simulink model "ackerman_ROS_neural_controller_v2"  (R2023a)
settings: Solver=FixedStepDiscrete  StartTime=0.0  StopTime=200  FixedStep=0.1  RelTol=1e-3
undefined symbols (not defined in the file or in its folder): Angular, Linear
libraries: neural x413, robotlib x15, robotcorelib x1
(part 4 of 17)

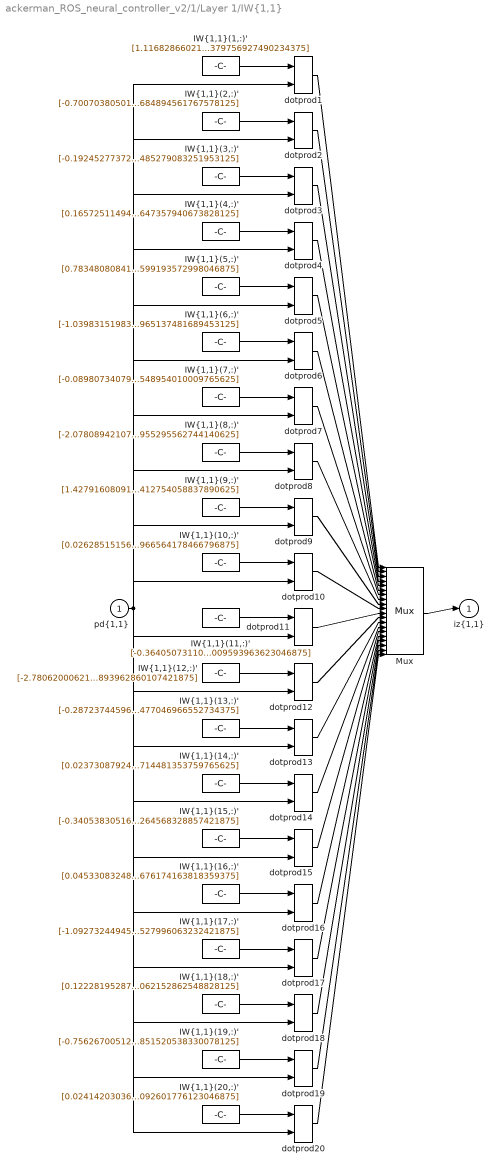
== system ackerman_ROS_neural_controller_v2/1/Layer 1/IW{1,1} ==
  "pd{1,1}" : Inport  PortDimensions=8  SampleTime=0.1
      mask Display: e = 0.06;c1 = [120 230 180]/255;c2 = ([120 230 180]+0)/(256+128);c3 = ([120 230 180]+128)/(256+128);patch([0 1 1 0],[0 0 1 1],c1);patch([0 1 1 1-e 1-e 0+e],[0 0 1 1-e 0+e 0+e],c2);patch([0 0 1 1-e 0+e 0+e],[0 1 1 1-e 1-e 0+e],c3);plot([0 1 1 0 0],[0 0 1 1 0]);
  "IW{1,1}(1,:)'" : Constant  Value=[1.116828660219907565220864853472448885440826416015625;-1.317372152173824861876028080587275326251983642578125;0.0888240780158889020601264974175137467682361602783203125;0.811843799445297609196359189809300005435943603515625;-0.0697394502326299237093820693189627490937709808349609375;-0.9124948278432263304438265549833886325359344482421875;0.48823599511569326647730804324964992702007293701171875;0.92312336239510184299206230207346379756927490234375]
      mask Display: e = 0.06;c1 = [120 150 230]/255;c2 = ([120 150 230]+0)/383;c3 = ([120 150 230]+128)/383;patch([0 1 1 0],[0 0 1 1],c1);patch([0 1 1 1-e 1-e 0+e],[0 0 1 1-e 0+e 0+e],c2);patch([0 0 1 1-e 0+e 0+e],[0 1 1 1-e 1-e 0+e],c3);plot([0 1 1 0 0],[0 0 1 1 0]);disp('Weights');
  "IW{1,1}(10,:)'" : Constant  Value=[0.0262851515602594322518203995286967256106436252593994140625;-2.5598472339347626558492265758104622364044189453125;-0.63500001320806076510194770889938808977603912353515625;0.08080628574030923605420184685499407351016998291015625;0.004282547131209214763547521442887955345213413238525390625;0.18751429268016039930699889737297780811786651611328125;0.50378156376655447434842471921001560986042022705078125;-0.52232179336882456066604163424926809966564178466796875]
      mask Display: e = 0.06;c1 = [120 150 230]/255;c2 = ([120 150 230]+0)/383;c3 = ([120 150 230]+128)/383;patch([0 1 1 0],[0 0 1 1],c1);patch([0 1 1 1-e 1-e 0+e],[0 0 1 1-e 0+e 0+e],c2);patch([0 0 1 1-e 0+e 0+e],[0 1 1 1-e 1-e 0+e],c3);plot([0 1 1 0 0],[0 0 1 1 0]);disp('Weights');
  "IW{1,1}(11,:)'" : Constant  Value=[-0.364050731103570779367828436079435050487518310546875;1.8340052162234459220968574300059117376804351806640625;0.0010169610273991704259277657484972223755903542041778564453125;0.58347480564712761452739187006955035030841827392578125;-0.9371891608231053272248800567467696964740753173828125;-0.721163434606463482623439631424844264984130859375;2.035079423445592450292451758286915719509124755859375;-0.34513579930387716654394125725957565009593963623046875]
      mask Display: e = 0.06;c1 = [120 150 230]/255;c2 = ([120 150 230]+0)/383;c3 = ([120 150 230]+128)/383;patch([0 1 1 0],[0 0 1 1],c1);patch([0 1 1 1-e 1-e 0+e],[0 0 1 1-e 0+e 0+e],c2);patch([0 0 1 1-e 0+e 0+e],[0 1 1 1-e 1-e 0+e],c3);plot([0 1 1 0 0],[0 0 1 1 0]);disp('Weights');
  "IW{1,1}(12,:)'" : Constant  Value=[-2.78062000621869831462618094519712030887603759765625;1.121862788646456277064089590567164123058319091796875;-1.8782585151834967351902605514624156057834625244140625;-1.8760642857863503163429186315624974668025970458984375;0.63081995495714615618254583750967867672443389892578125;1.7257064609143097921872822553268633782863616943359375;0.1502900196201445714994093805216834880411624908447265625;1.2290305602665305695353481496567837893962860107421875]
      mask Display: e = 0.06;c1 = [120 150 230]/255;c2 = ([120 150 230]+0)/383;c3 = ([120 150 230]+128)/383;patch([0 1 1 0],[0 0 1 1],c1);patch([0 1 1 1-e 1-e 0+e],[0 0 1 1-e 0+e 0+e],c2);patch([0 0 1 1-e 0+e 0+e],[0 1 1 1-e 1-e 0+e],c3);plot([0 1 1 0 0],[0 0 1 1 0]);disp('Weights');
  "IW{1,1}(13,:)'" : Constant  Value=[-0.2872374459617628161822722177021205425262451171875;-2.905786860043843233825100469402968883514404296875;-0.553996651955559027413755757152102887630462646484375;0.86810930276092801438636570310336537659168243408203125;-0.73141176276367680930690085006062872707843780517578125;0.687679406082589483872880009585060179233551025390625;0.1435056389676894472717805228967336006462574005126953125;-0.098326242430082311241079651153995655477046966552734375]
      mask Display: e = 0.06;c1 = [120 150 230]/255;c2 = ([120 150 230]+0)/383;c3 = ([120 150 230]+128)/383;patch([0 1 1 0],[0 0 1 1],c1);patch([0 1 1 1-e 1-e 0+e],[0 0 1 1-e 0+e 0+e],c2);patch([0 0 1 1-e 0+e 0+e],[0 1 1 1-e 1-e 0+e],c3);plot([0 1 1 0 0],[0 0 1 1 0]);disp('Weights');
  "IW{1,1}(14,:)'" : Constant  Value=[0.0237308792477848133628537397044055978767573833465576171875;-1.601784995976378578319554435438476502895355224609375;0.405350870218719183668554251198656857013702392578125;-0.007838045313262813340582368937248247675597667694091796875;0.32434432315157002424399479423300363123416900634765625;-1.0640785119557130133927103088353760540485382080078125;1.5009538196627640882496734775486402213573455810546875;-0.088510228652192657339270454031066037714481353759765625]
      mask Display: e = 0.06;c1 = [120 150 230]/255;c2 = ([120 150 230]+0)/383;c3 = ([120 150 230]+128)/383;patch([0 1 1 0],[0 0 1 1],c1);patch([0 1 1 1-e 1-e 0+e],[0 0 1 1-e 0+e 0+e],c2);patch([0 0 1 1-e 0+e 0+e],[0 1 1 1-e 1-e 0+e],c3);plot([0 1 1 0 0],[0 0 1 1 0]);disp('Weights');
  "IW{1,1}(15,:)'" : Constant  Value=[-0.3405383051671406757776594531605951488018035888671875;0.053295252358578293350177546017221175134181976318359375;1.035586391719500287678101813071407377719879150390625;1.923473416234176891492779759573750197887420654296875;-0.277425310964073024155851499017444439232349395751953125;-1.072290053858897973526609348482452332973480224609375;0.8387550177294522679716237689717672765254974365234375;-1.3760015689854945275527597914333455264568328857421875]
      mask Display: e = 0.06;c1 = [120 150 230]/255;c2 = ([120 150 230]+0)/383;c3 = ([120 150 230]+128)/383;patch([0 1 1 0],[0 0 1 1],c1);patch([0 1 1 1-e 1-e 0+e],[0 0 1 1-e 0+e 0+e],c2);patch([0 0 1 1-e 0+e 0+e],[0 1 1 1-e 1-e 0+e],c3);plot([0 1 1 0 0],[0 0 1 1 0]);disp('Weights');
  "IW{1,1}(16,:)'" : Constant  Value=[0.0453308324853925193043124863834236748516559600830078125;0.459559343539199749439916331539279781281948089599609375;-1.5227217158325867529811148415319621562957763671875;-0.6914425749720829461608673227601684629917144775390625;0.4436755063765982498580342507921159267425537109375;0.455038286792085522325379542962764389812946319580078125;0.9115280177617386403454702303861267864704132080078125;0.82498647477164011032613188945106230676174163818359375]
      mask Display: e = 0.06;c1 = [120 150 230]/255;c2 = ([120 150 230]+0)/383;c3 = ([120 150 230]+128)/383;patch([0 1 1 0],[0 0 1 1],c1);patch([0 1 1 1-e 1-e 0+e],[0 0 1 1-e 0+e 0+e],c2);patch([0 0 1 1-e 0+e 0+e],[0 1 1 1-e 1-e 0+e],c3);plot([0 1 1 0 0],[0 0 1 1 0]);disp('Weights');
  "IW{1,1}(17,:)'" : Constant  Value=[-1.0927324494595291870524533806019462645053863525390625;0.1538524822892356203052344199022627435624599456787109375;0.0671074562694427279030406907622818835079669952392578125;-0.57349675474466821345487232974846847355365753173828125;1.6003783061698844125686491679516620934009552001953125;1.60480486204609018585642843390814960002899169921875;-0.50380125898334504608300221661920659244060516357421875;0.59042401286813450678181425246293656527996063232421875]
      mask Display: e = 0.06;c1 = [120 150 230]/255;c2 = ([120 150 230]+0)/383;c3 = ([120 150 230]+128)/383;patch([0 1 1 0],[0 0 1 1],c1);patch([0 1 1 1-e 1-e 0+e],[0 0 1 1-e 0+e 0+e],c2);patch([0 0 1 1-e 0+e 0+e],[0 1 1 1-e 1-e 0+e],c3);plot([0 1 1 0 0],[0 0 1 1 0]);disp('Weights');
  "IW{1,1}(18,:)'" : Constant  Value=[0.12228195287823399872717544667466427199542522430419921875;-0.354406976130497763932680754805915057659149169921875;1.16787670361109707783953126636333763599395751953125;-0.171791758447963960332316446510958485305309295654296875;-0.7120100985359341105862540644011460244655609130859375;-1.0292471435836361148830064848880283534526824951171875;-1.6915065806122473457406840680050663650035858154296875;0.2143675751442244703515171977414865978062152862548828125]
      mask Display: e = 0.06;c1 = [120 150 230]/255;c2 = ([120 150 230]+0)/383;c3 = ([120 150 230]+128)/383;patch([0 1 1 0],[0 0 1 1],c1);patch([0 1 1 1-e 1-e 0+e],[0 0 1 1-e 0+e 0+e],c2);patch([0 0 1 1-e 0+e 0+e],[0 1 1 1-e 1-e 0+e],c3);plot([0 1 1 0 0],[0 0 1 1 0]);disp('Weights');
  "IW{1,1}(19,:)'" : Constant  Value=[-0.7562670051233231216514241168624721467494964599609375;-0.85460135528397873638795090300845913589000701904296875;0.85019606027952299154293314131791703402996063232421875;0.1161628518467531512303736462854431010782718658447265625;-1.0109441109467194319648797318222932517528533935546875;-0.94125834497824223401352128348662517964839935302734375;-0.794270812434147988057020484120585024356842041015625;-0.3913546009844559581125622571562416851520538330078125]
      mask Display: e = 0.06;c1 = [120 150 230]/255;c2 = ([120 150 230]+0)/383;c3 = ([120 150 230]+128)/383;patch([0 1 1 0],[0 0 1 1],c1);patch([0 1 1 1-e 1-e 0+e],[0 0 1 1-e 0+e 0+e],c2);patch([0 0 1 1-e 0+e 0+e],[0 1 1 1-e 1-e 0+e],c3);plot([0 1 1 0 0],[0 0 1 1 0]);disp('Weights');
  "IW{1,1}(2,:)'" : Constant  Value=[-0.70070380501134021944409369098138995468616485595703125;0.4463782749714180209110736541333608329296112060546875;0.67982390187422991889576451285392977297306060791015625;-0.66805266049382705517700742348097264766693115234375;0.65873385787125737778069378691725432872772216796875;0.80873570737898192728465573964058421552181243896484375;1.607933726033231369711984370951540768146514892578125;0.0282312561074684886808228156951372511684894561767578125]
      mask Display: e = 0.06;c1 = [120 150 230]/255;c2 = ([120 150 230]+0)/383;c3 = ([120 150 230]+128)/383;patch([0 1 1 0],[0 0 1 1],c1);patch([0 1 1 1-e 1-e 0+e],[0 0 1 1-e 0+e 0+e],c2);patch([0 0 1 1-e 0+e 0+e],[0 1 1 1-e 1-e 0+e],c3);plot([0 1 1 0 0],[0 0 1 1 0]);disp('Weights');
  "IW{1,1}(20,:)'" : Constant  Value=[0.0241420303636170376082592525790460058487951755523681640625;-0.222720935580721646207535968642332591116428375244140625;0.323902677318082365953699763849726878106594085693359375;-0.6235037611809357560588296109926886856555938720703125;-0.69145330685383232793839169971761293709278106689453125;-1.0351207523282039968393064555129967629909515380859375;0.365678623892759235847194076995947398245334625244140625;-2.616536737179383731444204386207275092601776123046875]
      mask Display: e = 0.06;c1 = [120 150 230]/255;c2 = ([120 150 230]+0)/383;c3 = ([120 150 230]+128)/383;patch([0 1 1 0],[0 0 1 1],c1);patch([0 1 1 1-e 1-e 0+e],[0 0 1 1-e 0+e 0+e],c2);patch([0 0 1 1-e 0+e 0+e],[0 1 1 1-e 1-e 0+e],c3);plot([0 1 1 0 0],[0 0 1 1 0]);disp('Weights');
  "IW{1,1}(3,:)'" : Constant  Value=[-0.1924527737266698290685695837964885868132114410400390625;-0.98526738913007749776085120174684561789035797119140625;1.182387309836708144672456910484470427036285400390625;0.140201368902994116805160729199997149407863616943359375;-1.784628432745574588835779650253243744373321533203125;0.8833279993245153338676800558459945023059844970703125;0.8505388438650627325188224858720786869525909423828125;-0.331496701624171496991522190000978298485279083251953125]
      mask Display: e = 0.06;c1 = [120 150 230]/255;c2 = ([120 150 230]+0)/383;c3 = ([120 150 230]+128)/383;patch([0 1 1 0],[0 0 1 1],c1);patch([0 1 1 1-e 1-e 0+e],[0 0 1 1-e 0+e 0+e],c2);patch([0 0 1 1-e 0+e 0+e],[0 1 1 1-e 1-e 0+e],c3);plot([0 1 1 0 0],[0 0 1 1 0]);disp('Weights');
  "IW{1,1}(4,:)'" : Constant  Value=[0.1657251149471581086469740284883300773799419403076171875;0.11079163994764328060593783220610930584371089935302734375;1.1628412946805528616067704206216149032115936279296875;1.3120470595789817114251718521700240671634674072265625;0.5705449810256768561345097623416222631931304931640625;0.2195264626413448161290631333031342364847660064697265625;-2.660419563695247457957293590879999101161956787109375;-0.7954052280397139185197374899871647357940673828125]
      mask Display: e = 0.06;c1 = [120 150 230]/255;c2 = ([120 150 230]+0)/383;c3 = ([120 150 230]+128)/383;patch([0 1 1 0],[0 0 1 1],c1);patch([0 1 1 1-e 1-e 0+e],[0 0 1 1-e 0+e 0+e],c2);patch([0 0 1 1-e 0+e 0+e],[0 1 1 1-e 1-e 0+e],c3);plot([0 1 1 0 0],[0 0 1 1 0]);disp('Weights');
  "IW{1,1}(5,:)'" : Constant  Value=[0.7834808084145892248528753043501637876033782958984375;-1.42447445469726829969658865593373775482177734375;1.1975312359302596743049207361764274537563323974609375;0.1635490607498303050615362508324324153363704681396484375;-0.6718969042920146517161583687993697822093963623046875;-0.1372657172031984396110004809088422916829586029052734375;0.38125925588003173327678041459876112639904022216796875;-1.4402596893604620031936747182044200599193572998046875]
      mask Display: e = 0.06;c1 = [120 150 230]/255;c2 = ([120 150 230]+0)/383;c3 = ([120 150 230]+128)/383;patch([0 1 1 0],[0 0 1 1],c1);patch([0 1 1 1-e 1-e 0+e],[0 0 1 1-e 0+e 0+e],c2);patch([0 0 1 1-e 0+e 0+e],[0 1 1 1-e 1-e 0+e],c3);plot([0 1 1 0 0],[0 0 1 1 0]);disp('Weights');
  "IW{1,1}(6,:)'" : Constant  Value=[-1.0398315198302390260920446962700225412845611572265625;1.0759366572930788574780081034987233579158782958984375;-0.180033990146306888124883016644162125885486602783203125;-1.348012567824036889163608066155575215816497802734375;-2.885573301576848326277513478999026119709014892578125;-0.2948558223190076432729256339371204376220703125;1.2807460752471115927875189299811609089374542236328125;0.08268843179290515099655323183469590730965137481689453125]
      mask Display: e = 0.06;c1 = [120 150 230]/255;c2 = ([120 150 230]+0)/383;c3 = ([120 150 230]+128)/383;patch([0 1 1 0],[0 0 1 1],c1);patch([0 1 1 1-e 1-e 0+e],[0 0 1 1-e 0+e 0+e],c2);patch([0 0 1 1-e 0+e 0+e],[0 1 1 1-e 1-e 0+e],c3);plot([0 1 1 0 0],[0 0 1 1 0]);disp('Weights');
  "IW{1,1}(7,:)'" : Constant  Value=[-0.08980734079662848479141956659077550284564495086669921875;-0.1641338178963755167760751874084235168993473052978515625;0.405589455292452161216942840837873518466949462890625;1.076734142043771047525524409138597548007965087890625;0.54123529493598188100378365561482496559619903564453125;1.1029221929994712514400134750758297741413116455078125;1.648597514590885548813048444571904838085174560546875;-1.5057803317372295826004346963600255548954010009765625]
      mask Display: e = 0.06;c1 = [120 150 230]/255;c2 = ([120 150 230]+0)/383;c3 = ([120 150 230]+128)/383;patch([0 1 1 0],[0 0 1 1],c1);patch([0 1 1 1-e 1-e 0+e],[0 0 1 1-e 0+e 0+e],c2);patch([0 0 1 1-e 0+e 0+e],[0 1 1 1-e 1-e 0+e],c3);plot([0 1 1 0 0],[0 0 1 1 0]);disp('Weights');
  "IW{1,1}(8,:)'" : Constant  Value=[-2.07808942107180172342850710265338420867919921875;-1.0129688078326017919295054525719024240970611572265625;0.275033497576107344162466006309841759502887725830078125;0.48072637579094390503087197430431842803955078125;-0.023912142949013927284429570363499806262552738189697265625;0.5059355504927471880449729724205099046230316162109375;-0.46415439958115023433293799826060421764850616455078125;2.02330328464420805545387338497675955295562744140625]
      mask Display: e = 0.06;c1 = [120 150 230]/255;c2 = ([120 150 230]+0)/383;c3 = ([120 150 230]+128)/383;patch([0 1 1 0],[0 0 1 1],c1);patch([0 1 1 1-e 1-e 0+e],[0 0 1 1-e 0+e 0+e],c2);patch([0 0 1 1-e 0+e 0+e],[0 1 1 1-e 1-e 0+e],c3);plot([0 1 1 0 0],[0 0 1 1 0]);disp('Weights');
  "IW{1,1}(9,:)'" : Constant  Value=[1.4279160809158355505132931284606456756591796875;-1.035532835891061598232454343815334141254425048828125;-0.5968860108683367027282429262413643300533294677734375;-1.2494838793611282579121279923128895461559295654296875;3.934956615032649818175514155882410705089569091796875;0.1307241221935328268077824986903578974306583404541015625;-2.457926598366699355580067276605404913425445556640625;-1.627164141237702921216623508371412754058837890625]
      mask Display: e = 0.06;c1 = [120 150 230]/255;c2 = ([120 150 230]+0)/383;c3 = ([120 150 230]+128)/383;patch([0 1 1 0],[0 0 1 1],c1);patch([0 1 1 1-e 1-e 0+e],[0 0 1 1-e 0+e 0+e],c2);patch([0 0 1 1-e 0+e 0+e],[0 1 1 1-e 1-e 0+e],c3);plot([0 1 1 0 0],[0 0 1 1 0]);disp('Weights');
  Mux : Mux  Inputs=20
      mask Display: e = 0.06;c1 = [120 150 230]/255;c2 = ([120 150 230]+0)/383;c3 = ([120 150 230]+128)/383;patch([0 1 1 0],[0 0 1 1],c1);patch([0 1 1 1-e 1-e 0+e],[0 0 1 1-e 0+e 0+e],c2);patch([0 0 1 1-e 0+e 0+e],[0 1 1 1-e 1-e 0+e],c3);plot([0 1 1 0 0],[0 0 1 1 0]);disp('Mux');
  dotprod{1..20} (20 alike) : neural/Weight Functions/dotprod
  "iz{1,1}" : Outport
      mask Display: e = 0.06;c1 = [120 230 180]/255;c2 = ([120 230 180]+0)/(256+128);c3 = ([120 230 180]+128)/(256+128);patch([0 1 1 0],[0 0 1 1],c1);patch([0 1 1 1-e 1-e 0+e],[0 0 1 1-e 0+e 0+e],c2);patch([0 0 1 1-e 0+e 0+e],[0 1 1 1-e 1-e 0+e],c3);plot([0 1 1 0 0],[0 0 1 1 0]);
  wires:
  "IW{1,1}(1,:)'"/1 -> dotprod1/1
  "pd{1,1}"/1 -> dotprod1/2, dotprod2/2, dotprod3/2, dotprod4/2, dotprod5/2, dotprod6/2, dotprod7/2, dotprod8/2, dotprod9/2, dotprod10/2, dotprod11/2, dotprod12/2, dotprod13/2, dotprod14/2, dotprod15/2, dotprod16/2, dotprod17/2, dotprod18/2, dotprod19/2, dotprod20/2
  dotprod1/1 -> Mux/1
  "IW{1,1}(2,:)'"/1 -> dotprod2/1
  dotprod2/1 -> Mux/2
  "IW{1,1}(3,:)'"/1 -> dotprod3/1
  dotprod3/1 -> Mux/3
  "IW{1,1}(4,:)'"/1 -> dotprod4/1
  dotprod4/1 -> Mux/4
  "IW{1,1}(5,:)'"/1 -> dotprod5/1
  dotprod5/1 -> Mux/5
  "IW{1,1}(6,:)'"/1 -> dotprod6/1
  dotprod6/1 -> Mux/6
  "IW{1,1}(7,:)'"/1 -> dotprod7/1
  dotprod7/1 -> Mux/7
  "IW{1,1}(8,:)'"/1 -> dotprod8/1
  dotprod8/1 -> Mux/8
  "IW{1,1}(9,:)'"/1 -> dotprod9/1
  dotprod9/1 -> Mux/9
  "IW{1,1}(10,:)'"/1 -> dotprod10/1
  dotprod10/1 -> Mux/10
  "IW{1,1}(11,:)'"/1 -> dotprod11/1
  dotprod11/1 -> Mux/11
  "IW{1,1}(12,:)'"/1 -> dotprod12/1
  dotprod12/1 -> Mux/12
  "IW{1,1}(13,:)'"/1 -> dotprod13/1
  dotprod13/1 -> Mux/13
  "IW{1,1}(14,:)'"/1 -> dotprod14/1
  dotprod14/1 -> Mux/14
  "IW{1,1}(15,:)'"/1 -> dotprod15/1
  dotprod15/1 -> Mux/15
  "IW{1,1}(16,:)'"/1 -> dotprod16/1
  dotprod16/1 -> Mux/16
  "IW{1,1}(17,:)'"/1 -> dotprod17/1
  dotprod17/1 -> Mux/17
  "IW{1,1}(18,:)'"/1 -> dotprod18/1
  dotprod18/1 -> Mux/18
  "IW{1,1}(19,:)'"/1 -> dotprod19/1
  dotprod19/1 -> Mux/19
  "IW{1,1}(20,:)'"/1 -> dotprod20/1
  dotprod20/1 -> Mux/20
  Mux/1 -> "iz{1,1}"/1

== system ackerman_ROS_neural_controller_v2/1/Layer 2/Delays 1 ==
  "p{2}" : Inport  PortDimensions=20  SampleTime=0.1
      mask Display: e = 0.06;c1 = [120 230 180]/255;c2 = ([120 230 180]+0)/(256+128);c3 = ([120 230 180]+128)/(256+128);patch([0 1 1 0],[0 0 1 1],c1);patch([0 1 1 1-e 1-e 0+e],[0 0 1 1-e 0+e 0+e],c2);patch([0 0 1 1-e 0+e 0+e],[0 1 1 1-e 1-e 0+e],c3);plot([0 1 1 0 0],[0 0 1 1 0]);
  mux : Mux  Inputs=1
      mask Display: e = 0.06;c1 = [120 150 230]/255;c2 = ([120 150 230]+0)/383;c3 = ([120 150 230]+128)/383;patch([0 1 1 0],[0 0 1 1],c1);patch([0 1 1 1-e 1-e 0+e],[0 0 1 1-e 0+e 0+e],c2);patch([0 0 1 1-e 0+e 0+e],[0 1 1 1-e 1-e 0+e],c3);plot([0 1 1 0 0],[0 0 1 1 0]);disp('Mux')
  "pd{2,1}" : Outport
      mask Display: e = 0.06;c1 = [120 230 180]/255;c2 = ([120 230 180]+0)/(256+128);c3 = ([120 230 180]+128)/(256+128);patch([0 1 1 0],[0 0 1 1],c1);patch([0 1 1 1-e 1-e 0+e],[0 0 1 1-e 0+e 0+e],c2);patch([0 0 1 1-e 0+e 0+e],[0 1 1 1-e 1-e 0+e],c3);plot([0 1 1 0 0],[0 0 1 1 0]);
  wires:
  "p{2}"/1 -> mux/1
  mux/1 -> "pd{2,1}"/1

== system ackerman_ROS_neural_controller_v2/1/Layer 2/LW{2,1} ==
  "ad{2,1}" : Inport  PortDimensions=20  SampleTime=0.1
      mask Display: e = 0.06;c1 = [120 230 180]/255;c2 = ([120 230 180]+0)/(256+128);c3 = ([120 230 180]+128)/(256+128);patch([0 1 1 0],[0 0 1 1],c1);patch([0 1 1 1-e 1-e 0+e],[0 0 1 1-e 0+e 0+e],c2);patch([0 0 1 1-e 0+e 0+e],[0 1 1 1-e 1-e 0+e],c3);plot([0 1 1 0 0],[0 0 1 1 0]);
  "IW{2,1}(1,:)'" : Constant  Value=[0.110281640354253307467757849735789932310581207275390625;-0.4075499594610167974906289600767195224761962890625;-0.211945196756619658184916943355347029864788055419921875;-1.0447559407086106642026379631715826690196990966796875;0.99973827271722426335287536858231760561466217041015625;1.1187491991695612814083915509399957954883575439453125;-0.8574904128367728528559155165567062795162200927734375;-1.9045319663374866703264842726639471948146820068359375;2.507081512845534376765499473549425601959228515625;0.0009773874370581879522656976178041077218949794769287109375;0.1290398987580549661213780154866981320083141326904296875;-0.884324725107169751225910658831708133220672607421875;-0.448646363139221182603222359830397181212902069091796875;-0.5078166421618230952361727759125642478466033935546875;-1.0801208830190149878802685634582303464412689208984375;-0.220075278352753922472828662648680619895458221435546875;0.1932052062463338604203499926370568573474884033203125;-0.268976457076010866398263488008524291217327117919921875;0.8706129490286713679125796261359937489032745361328125;-0.12354111103369637414406412290190928615629673004150390625]
      mask Display: e = 0.06;c1 = [120 150 230]/255;c2 = ([120 150 230]+0)/383;c3 = ([120 150 230]+128)/383;patch([0 1 1 0],[0 0 1 1],c1);patch([0 1 1 1-e 1-e 0+e],[0 0 1 1-e 0+e 0+e],c2);patch([0 0 1 1-e 0+e 0+e],[0 1 1 1-e 1-e 0+e],c3);plot([0 1 1 0 0],[0 0 1 1 0]);disp('weights');
  "IW{2,1}(10,:)'" : Constant  Value=[0.346280781819803429311122044964577071368694305419921875;0.064764388127894034763443187330267392098903656005859375;-0.198841117778091935885953489560051821172237396240234375;-0.1526219736868450194133828290432575158774852752685546875;-0.315671952489745388792385938359075225889682769775390625;0.41149032816694230962895062475581653416156768798828125;0.179963111618439197680885399677208624780178070068359375;-0.6692435375154885957016404063324443995952606201171875;-0.69612096619450680723417690387577749788761138916015625;-0.42825439692942079972226565587334334850311279296875;0.041563970098095683047834114631768898107111454010009765625;-0.1601867703146730714802714601319166831672191619873046875;0.6738085909001958473396598492399789392948150634765625;0.1940185562231697968815780086515587754547595977783203125;-0.342702712650292451446176755780470557510852813720703125;0.74770586496094837425374635131447575986385345458984375;-0.25702064669828994514233500012778677046298980712890625;0.31617480897826855112953126081265509128570556640625;-0.24096465028794700202752210316248238086700439453125;-0.7483797507369989165937340658274479210376739501953125]
      mask Display: e = 0.06;c1 = [120 150 230]/255;c2 = ([120 150 230]+0)/383;c3 = ([120 150 230]+128)/383;patch([0 1 1 0],[0 0 1 1],c1);patch([0 1 1 1-e 1-e 0+e],[0 0 1 1-e 0+e 0+e],c2);patch([0 0 1 1-e 0+e 0+e],[0 1 1 1-e 1-e 0+e],c3);plot([0 1 1 0 0],[0 0 1 1 0]);disp('weights');
  "IW{2,1}(2,:)'" : Constant  Value=[-0.3144161658093695965732194963493384420871734619140625;-0.260802005499317868242314943927340209484100341796875;-0.09118866387487238600595418347438680939376354217529296875;-0.1779746583379019087001182697349577210843563079833984375;0.273944070348914270329743203546968288719654083251953125;0.1429879515740476170204686923170811496675014495849609375;-0.353011636830328157099501140692154876887798309326171875;-0.48203732900629636670686295474297367036342620849609375;-0.5762308390680572767195144479046575725078582763671875;-0.147680072840977005821372358695953153073787689208984375;-0.351694320118391690055403842052328400313854217529296875;-0.12110239440517685249876222997045260854065418243408203125;-0.1729993563477275342332717400495312176644802093505859375;-0.2449324314496446886035840861950418911874294281005859375;0.290852554535415308567536385453422553837299346923828125;0.48214156352169867947310422096052207052707672119140625;-0.1768665440642207264954066658901865594089031219482421875;-0.6433962295717943202788546841475181281566619873046875;-0.61118602203887972823537211297661997377872467041015625;-0.64264309517045792308209684051689691841602325439453125]
      mask Display: e = 0.06;c1 = [120 150 230]/255;c2 = ([120 150 230]+0)/383;c3 = ([120 150 230]+128)/383;patch([0 1 1 0],[0 0 1 1],c1);patch([0 1 1 1-e 1-e 0+e],[0 0 1 1-e 0+e 0+e],c2);patch([0 0 1 1-e 0+e 0+e],[0 1 1 1-e 1-e 0+e],c3);plot([0 1 1 0 0],[0 0 1 1 0]);disp('weights');
  "IW{2,1}(3,:)'" : Constant  Value=[-1.0531416570213278927070632562390528619289398193359375;0.021168604966173142079011171290403581224381923675537109375;-0.497619065788888426116187702064053155481815338134765625;-0.70600061911108136225578846278949640691280364990234375;-0.799145216720182904879266061470843851566314697265625;0.656441274846339073434364763670600950717926025390625;-1.0986685679554508698885229023289866745471954345703125;0.5647820076666738575710269287810660898685455322265625;1.2692212929800776866073874771245755255222320556640625;0.400332946434238723387721847757347859442234039306640625;-0.1089433289215561428964207379976869560778141021728515625;-1.818493460995366017840524364146403968334197998046875;-0.66180348114890608091087642605998553335666656494140625;-1.2170049059022656212647461870801635086536407470703125;0.8486535437562900963115453123464249074459075927734375;0.37739936148836650264826175771304406225681304931640625;1.2761023790039784930883115521282888948917388916015625;-1.396101663000505421763364211074076592922210693359375;0.05986777040123077153754849177857977338135242462158203125;-0.1085682225433008130099921118016936816275119781494140625]
      mask Display: e = 0.06;c1 = [120 150 230]/255;c2 = ([120 150 230]+0)/383;c3 = ([120 150 230]+128)/383;patch([0 1 1 0],[0 0 1 1],c1);patch([0 1 1 1-e 1-e 0+e],[0 0 1 1-e 0+e 0+e],c2);patch([0 0 1 1-e 0+e 0+e],[0 1 1 1-e 1-e 0+e],c3);plot([0 1 1 0 0],[0 0 1 1 0]);disp('weights');
  "IW{2,1}(4,:)'" : Constant  Value=[0.7802649519735174177270664586103521287441253662109375;-0.2171648780590997585004942038722219876945018768310546875;-0.2644108571941050644937831748393364250659942626953125;-0.2326443889087644045776670509440009482204914093017578125;-1.443034579947640505537265198654495179653167724609375;-1.650885089865213206650196298141963779926300048828125;0.5932390807268961285814157236018218100070953369140625;-0.423310015863895883203582570786238647997379302978515625;-0.7824745148668592609197958154254592955112457275390625;-1.0564054180223629852974909226759336888790130615234375;-0.48060704625918904131509634680696763098239898681640625;0.394917352231212548385741456513642333447933197021484375;-1.6965769318066958870616645072004757821559906005859375;-0.82689983880989059716881683925748802721500396728515625;-0.66916391659144658365931945809279568493366241455078125;-0.334444529874724338913694055008818395435810089111328125;-1.65208126900715246421214033034630119800567626953125;1.364022987750377335913753995555453002452850341796875;-0.0093443227721153702958201137107607792131602764129638671875;-0.56926038307607884636496464736410416662693023681640625]
      mask Display: e = 0.06;c1 = [120 150 230]/255;c2 = ([120 150 230]+0)/383;c3 = ([120 150 230]+128)/383;patch([0 1 1 0],[0 0 1 1],c1);patch([0 1 1 1-e 1-e 0+e],[0 0 1 1-e 0+e 0+e],c2);patch([0 0 1 1-e 0+e 0+e],[0 1 1 1-e 1-e 0+e],c3);plot([0 1 1 0 0],[0 0 1 1 0]);disp('weights');
  "IW{2,1}(5,:)'" : Constant  Value=[-1.69558095268002251287953185965307056903839111328125;-0.036402227108619421291901829818016267381608486175537109375;0.79510630105207347195772626946563832461833953857421875;1.288678002327857452513626412837766110897064208984375;0.50338188136540684691766500691301189363002777099609375;0.0718388753007755120894017863975022919476032257080078125;0.89626959568035380332418071702704764902591705322265625;-1.545785879539742335708751852507703006267547607421875;-0.94793395213213982319899741924018599092960357666015625;1.225767400049665223349393272656016051769256591796875;-0.1410385296484627792867883044891641475260257720947265625;-2.26987855069070310065626472351141273975372314453125;0.82063433795832640971212867952999658882617950439453125;0.5657515729250663927274445086368359625339508056640625;1.474012242783430348680440147290937602519989013671875;0.638039091111959777435913565568625926971435546875;-0.6381713375893458550791592642781324684619903564453125;-1.1708364908966777395704639275209046900272369384765625;-0.19528457479245509009757597596035338938236236572265625;-0.6839118851799159681803530475008301436901092529296875]
      mask Display: e = 0.06;c1 = [120 150 230]/255;c2 = ([120 150 230]+0)/383;c3 = ([120 150 230]+128)/383;patch([0 1 1 0],[0 0 1 1],c1);patch([0 1 1 1-e 1-e 0+e],[0 0 1 1-e 0+e 0+e],c2);patch([0 0 1 1-e 0+e 0+e],[0 1 1 1-e 1-e 0+e],c3);plot([0 1 1 0 0],[0 0 1 1 0]);disp('weights');
  "IW{2,1}(6,:)'" : Constant  Value=[0.323379113562345665844333097993512637913227081298828125;0.63603235307997330050255868627573363482952117919921875;0.9136038407711459807813980660284869372844696044921875;-0.56666095330895605020060656897840090095996856689453125;0.159876383499391316878046609417651779949665069580078125;0.62063551392938454132064407531288452446460723876953125;0.2516353424530215487919804218108765780925750732421875;-0.104656037316503469636330692082992754876613616943359375;2.097313473759132573803753984975628554821014404296875;0.07834531276352570128285179862359655089676380157470703125;2.195634643091262550029796329909004271030426025390625;-1.3286965266555343934129496119567193090915679931640625;1.46608549856063330452116133528761565685272216796875;-0.88004902451046318478944385788054205477237701416015625;0.7740781740302422608834831407875753939151763916015625;-0.37138408893100860463931667254655621945858001708984375;1.604442288304878783122831009677611291408538818359375;-0.449110542112181210239185702448594383895397186279296875;0.06659377782630350461889889857047819532454013824462890625;-0.6823935781906842468202967211254872381687164306640625]
      mask Display: e = 0.06;c1 = [120 150 230]/255;c2 = ([120 150 230]+0)/383;c3 = ([120 150 230]+128)/383;patch([0 1 1 0],[0 0 1 1],c1);patch([0 1 1 1-e 1-e 0+e],[0 0 1 1-e 0+e 0+e],c2);patch([0 0 1 1-e 0+e 0+e],[0 1 1 1-e 1-e 0+e],c3);plot([0 1 1 0 0],[0 0 1 1 0]);disp('weights');
  "IW{2,1}(7,:)'" : Constant  Value=[0.32539695260053724812365771867916919291019439697265625;1.0963993598379910832107952955993823707103729248046875;-1.330554666607169256309362026513554155826568603515625;0.442056302963367897529423089508782140910625457763671875;0.82216341442806761818928862339816987514495849609375;-0.30352716797758072519997085692011751234531402587890625;0.2136723848484809451520050060935318470001220703125;-0.84521000613493135755760476968134753406047821044921875;-0.474420040044124025069294248169171623885631561279296875;-0.65302179764648382587211017380468547344207763671875;-0.106792482967198620880111548103741370141506195068359375;-0.004261715654998519953178259811465977691113948822021484375;-0.45342284495086493389948145704693160951137542724609375;-0.44167171573887176183603742174454964697360992431640625;0.054384844545579659469414224304273375310003757476806640625;-0.2631948573202540497817381037748418748378753662109375;-0.91589517807826392736814113959553651511669158935546875;-0.298081126093376891361685920855961740016937255859375;-0.00160608898792290850053576800604560048668645322322845458984375;-0.7363276965989420386193842205102555453777313232421875]
      mask Display: e = 0.06;c1 = [120 150 230]/255;c2 = ([120 150 230]+0)/383;c3 = ([120 150 230]+128)/383;patch([0 1 1 0],[0 0 1 1],c1);patch([0 1 1 1-e 1-e 0+e],[0 0 1 1-e 0+e 0+e],c2);patch([0 0 1 1-e 0+e 0+e],[0 1 1 1-e 1-e 0+e],c3);plot([0 1 1 0 0],[0 0 1 1 0]);disp('weights');
  "IW{2,1}(8,:)'" : Constant  Value=[0.32874612828760485516710332376533187925815582275390625;0.0710020987546251536315367047791369259357452392578125;1.4334982317991258327083414769731462001800537109375;-1.64361634671000000906815330381505191326141357421875;1.2149991778035751366360273095779120922088623046875;-0.394753699083970122085673892797785811126232147216796875;0.9532826631658524174639524062513373792171478271484375;1.0760849088790676031379689447931014001369476318359375;0.37104541140617808281376710510812699794769287109375;-1.4184456485779743939446007061633281409740447998046875;-0.620210822933957128810789072304032742977142333984375;0.15774521529594431878962268456234596669673919677734375;-0.13276315570032470869676899383193813264369964599609375;-0.9063930202827121807018784238607622683048248291015625;0.1563201627598622411863260595055180601775646209716796875;-0.16544532948018753071295350309810601174831390380859375;0.1394618012108962690209779111683019436895847320556640625;-0.4205911415222323146423377693281508982181549072265625;0.004315684947857068194665419724742605467326939105987548828125;2.089247165072875223046366954804398119449615478515625]
      mask Display: e = 0.06;c1 = [120 150 230]/255;c2 = ([120 150 230]+0)/383;c3 = ([120 150 230]+128)/383;patch([0 1 1 0],[0 0 1 1],c1);patch([0 1 1 1-e 1-e 0+e],[0 0 1 1-e 0+e 0+e],c2);patch([0 0 1 1-e 0+e 0+e],[0 1 1 1-e 1-e 0+e],c3);plot([0 1 1 0 0],[0 0 1 1 0]);disp('weights');
  "IW{2,1}(9,:)'" : Constant  Value=[-0.1773281103387639723312219075523898936808109283447265625;0.54923976510526995031824526449781842529773712158203125;-0.1665812621925465697447776847184286452829837799072265625;0.50476248520914424045002988350461237132549285888671875;-1.1450841252226606759023752601933665573596954345703125;-0.298667354029940046444835388683713972568511962890625;-0.7945343766060466439427045770571567118167877197265625;-0.06821481375267528235450953388863126747310161590576171875;-0.05269335603690079861127770755047095008194446563720703125;0.25398566577575010239087305308203212916851043701171875;-0.2141097185808651104377275942169944755733013153076171875;-0.1355116118752296705540771881715045310556888580322265625;-0.1301537122175449312511119615010102279484272003173828125;0.11531863798625323347391002926087821833789348602294921875;-0.33685046075671232213011307976557873189449310302734375;0.75181738175153423053842516310396604239940643310546875;0.206085166155428378687020085635595023632049560546875;-0.7345387944372123723013601193088106811046600341796875;-0.52570409370548276672963083910872228443622589111328125;0.200735132107435543247220266493968665599822998046875]
      mask Display: e = 0.06;c1 = [120 150 230]/255;c2 = ([120 150 230]+0)/383;c3 = ([120 150 230]+128)/383;patch([0 1 1 0],[0 0 1 1],c1);patch([0 1 1 1-e 1-e 0+e],[0 0 1 1-e 0+e 0+e],c2);patch([0 0 1 1-e 0+e 0+e],[0 1 1 1-e 1-e 0+e],c3);plot([0 1 1 0 0],[0 0 1 1 0]);disp('weights');
  Mux : Mux  Inputs=10
      mask Display: e = 0.06;c1 = [120 150 230]/255;c2 = ([120 150 230]+0)/383;c3 = ([120 150 230]+128)/383;patch([0 1 1 0],[0 0 1 1],c1);patch([0 1 1 1-e 1-e 0+e],[0 0 1 1-e 0+e 0+e],c2);patch([0 0 1 1-e 0+e 0+e],[0 1 1 1-e 1-e 0+e],c3);plot([0 1 1 0 0],[0 0 1 1 0]);disp('Mux');
  dotprod{1..10} (10 alike) : neural/Weight Functions/dotprod
  "lz{2,1}" : Outport
      mask Display: e = 0.06;c1 = [120 230 180]/255;c2 = ([120 230 180]+0)/(256+128);c3 = ([120 230 180]+128)/(256+128);patch([0 1 1 0],[0 0 1 1],c1);patch([0 1 1 1-e 1-e 0+e],[0 0 1 1-e 0+e 0+e],c2);patch([0 0 1 1-e 0+e 0+e],[0 1 1 1-e 1-e 0+e],c3);plot([0 1 1 0 0],[0 0 1 1 0]);
  wires:
  "IW{2,1}(1,:)'"/1 -> dotprod1/1
  "ad{2,1}"/1 -> dotprod1/2, dotprod2/2, dotprod3/2, dotprod4/2, dotprod5/2, dotprod6/2, dotprod7/2, dotprod8/2, dotprod9/2, dotprod10/2
  dotprod1/1 -> Mux/1
  "IW{2,1}(2,:)'"/1 -> dotprod2/1
  dotprod2/1 -> Mux/2
  "IW{2,1}(3,:)'"/1 -> dotprod3/1
  dotprod3/1 -> Mux/3
  "IW{2,1}(4,:)'"/1 -> dotprod4/1
  dotprod4/1 -> Mux/4
  "IW{2,1}(5,:)'"/1 -> dotprod5/1
  dotprod5/1 -> Mux/5
  "IW{2,1}(6,:)'"/1 -> dotprod6/1
  dotprod6/1 -> Mux/6
  "IW{2,1}(7,:)'"/1 -> dotprod7/1
  dotprod7/1 -> Mux/7
  "IW{2,1}(8,:)'"/1 -> dotprod8/1
  dotprod8/1 -> Mux/8
  "IW{2,1}(9,:)'"/1 -> dotprod9/1
  dotprod9/1 -> Mux/9
  "IW{2,1}(10,:)'"/1 -> dotprod10/1
  dotprod10/1 -> Mux/10
  Mux/1 -> "lz{2,1}"/1

== system ackerman_ROS_neural_controller_v2/1/Layer 3/Delays 1 ==
  "p{3}" : Inport  PortDimensions=10  SampleTime=0.1
      mask Display: e = 0.06;c1 = [120 230 180]/255;c2 = ([120 230 180]+0)/(256+128);c3 = ([120 230 180]+128)/(256+128);patch([0 1 1 0],[0 0 1 1],c1);patch([0 1 1 1-e 1-e 0+e],[0 0 1 1-e 0+e 0+e],c2);patch([0 0 1 1-e 0+e 0+e],[0 1 1 1-e 1-e 0+e],c3);plot([0 1 1 0 0],[0 0 1 1 0]);
  mux : Mux  Inputs=1
      mask Display: e = 0.06;c1 = [120 150 230]/255;c2 = ([120 150 230]+0)/383;c3 = ([120 150 230]+128)/383;patch([0 1 1 0],[0 0 1 1],c1);patch([0 1 1 1-e 1-e 0+e],[0 0 1 1-e 0+e 0+e],c2);patch([0 0 1 1-e 0+e 0+e],[0 1 1 1-e 1-e 0+e],c3);plot([0 1 1 0 0],[0 0 1 1 0]);disp('Mux')
  "pd{3,2}" : Outport
      mask Display: e = 0.06;c1 = [120 230 180]/255;c2 = ([120 230 180]+0)/(256+128);c3 = ([120 230 180]+128)/(256+128);patch([0 1 1 0],[0 0 1 1],c1);patch([0 1 1 1-e 1-e 0+e],[0 0 1 1-e 0+e 0+e],c2);patch([0 0 1 1-e 0+e 0+e],[0 1 1 1-e 1-e 0+e],c3);plot([0 1 1 0 0],[0 0 1 1 0]);
  wires:
  "p{3}"/1 -> mux/1
  mux/1 -> "pd{3,2}"/1

== system ackerman_ROS_neural_controller_v2/1/Layer 3/LW{3,2} ==
  "ad{3,2}" : Inport  PortDimensions=10  SampleTime=0.1
      mask Display: e = 0.06;c1 = [120 230 180]/255;c2 = ([120 230 180]+0)/(256+128);c3 = ([120 230 180]+128)/(256+128);patch([0 1 1 0],[0 0 1 1],c1);patch([0 1 1 1-e 1-e 0+e],[0 0 1 1-e 0+e 0+e],c2);patch([0 0 1 1-e 0+e 0+e],[0 1 1 1-e 1-e 0+e],c3);plot([0 1 1 0 0],[0 0 1 1 0]);
  "IW{3,2}(1,:)'" : Constant  Value=[-0.890419222981996494326040192390792071819305419921875;-0.12460079972130444492250944676925428211688995361328125;-0.8858698531530979636272604693658649921417236328125;0.77487396696089039238586337887682020664215087890625;0.606830463136251996303371925023384392261505126953125;0.307909298698721245468590268501429818570613861083984375;-0.7598054481869549459105428468319587409496307373046875;0.7484997320190369674008934453013353049755096435546875;-0.633929518557385218713307040161453187465667724609375;0.0222909574330443505107979262902517803013324737548828125]
      mask Display: e = 0.06;c1 = [120 150 230]/255;c2 = ([120 150 230]+0)/383;c3 = ([120 150 230]+128)/383;patch([0 1 1 0],[0 0 1 1],c1);patch([0 1 1 1-e 1-e 0+e],[0 0 1 1-e 0+e 0+e],c2);patch([0 0 1 1-e 0+e 0+e],[0 1 1 1-e 1-e 0+e],c3);plot([0 1 1 0 0],[0 0 1 1 0]);disp('weights');
  "IW{3,2}(10,:)'" : Constant  Value=[-0.0206843812798684599518761473291306174360215663909912109375;-0.88992525516785991879231687562423758208751678466796875;-1.3830151728088131424243556466535665094852447509765625;0.287339427699368543667191033819108270108699798583984375;0.61871335592036602601950789903639815747737884521484375;0.6080998465495099924993382956017740070819854736328125;0.9506371002461218022716593623044900596141815185546875;-1.0638770603434564154810004765749908983707427978515625;0.22857555270375484735012605597148649394512176513671875;0.81076361606611102583741512717097066342830657958984375]
      mask Display: e = 0.06;c1 = [120 150 230]/255;c2 = ([120 150 230]+0)/383;c3 = ([120 150 230]+128)/383;patch([0 1 1 0],[0 0 1 1],c1);patch([0 1 1 1-e 1-e 0+e],[0 0 1 1-e 0+e 0+e],c2);patch([0 0 1 1-e 0+e 0+e],[0 1 1 1-e 1-e 0+e],c3);plot([0 1 1 0 0],[0 0 1 1 0]);disp('weights');
  "IW{3,2}(2,:)'" : Constant  Value=[0.6325799174656356882451291312463581562042236328125;-0.633033632287141045935641159303486347198486328125;-0.056581452627229543439479897415367304347455501556396484375;1.0014576633610590139511486995615996420383453369140625;-0.5878354486045742621769250035868026316165924072265625;0.270571808412681413802403085355763323605060577392578125;0.0304313569045785124733694004817152745090425014495849609375;0.61841711009884658967195036893826909363269805908203125;0.088651305674615044072339742342592217028141021728515625;-0.70742138270961885115895029230159707367420196533203125]
      mask Display: e = 0.06;c1 = [120 150 230]/255;c2 = ([120 150 230]+0)/383;c3 = ([120 150 230]+128)/383;patch([0 1 1 0],[0 0 1 1],c1);patch([0 1 1 1-e 1-e 0+e],[0 0 1 1-e 0+e 0+e],c2);patch([0 0 1 1-e 0+e 0+e],[0 1 1 1-e 1-e 0+e],c3);plot([0 1 1 0 0],[0 0 1 1 0]);disp('weights');
  "IW{3,2}(3,:)'" : Constant  Value=[0.459200104879947834657372141009545885026454925537109375;-1.250315345493625773798385125701315701007843017578125;-0.78895894862538373804028424274292774498462677001953125;-0.717057601658587895343544005299918353557586669921875;-0.61231648160025031746300783197511918842792510986328125;-0.86660957537572935738268142813467420637607574462890625;-0.2212265679656735539726497563606244511902332305908203125;0.491465527862171625006482145181507803499698638916015625;-1.03186574072127523749031752231530845165252685546875;-0.197849382377102589458672809996642172336578369140625]
      mask Display: e = 0.06;c1 = [120 150 230]/255;c2 = ([120 150 230]+0)/383;c3 = ([120 150 230]+128)/383;patch([0 1 1 0],[0 0 1 1],c1);patch([0 1 1 1-e 1-e 0+e],[0 0 1 1-e 0+e 0+e],c2);patch([0 0 1 1-e 0+e 0+e],[0 1 1 1-e 1-e 0+e],c3);plot([0 1 1 0 0],[0 0 1 1 0]);disp('weights');
  "IW{3,2}(4,:)'" : Constant  Value=[1.5189882959221616687273126444779336452484130859375;0.164683891109193181190306631833664141595363616943359375;0.22291202895959527641167596812010742723941802978515625;0.359589340705191384817140942686819471418857574462890625;-0.73054697529796819299718890761141665279865264892578125;0.446822583113995419612507475903839804232120513916015625;0.276599087912465180227883365660090930759906768798828125;-0.10942631039838392192908855804489576257765293121337890625;-0.1467577589642658220103754729279899038374423980712890625;0.70363986838549708036083529805182479321956634521484375]
      mask Display: e = 0.06;c1 = [120 150 230]/255;c2 = ([120 150 230]+0)/383;c3 = ([120 150 230]+128)/383;patch([0 1 1 0],[0 0 1 1],c1);patch([0 1 1 1-e 1-e 0+e],[0 0 1 1-e 0+e 0+e],c2);patch([0 0 1 1-e 0+e 0+e],[0 1 1 1-e 1-e 0+e],c3);plot([0 1 1 0 0],[0 0 1 1 0]);disp('weights');
  "IW{3,2}(5,:)'" : Constant  Value=[-0.106049464883745836463191380971693433821201324462890625;-0.98252510844313312166065088604227639734745025634765625;2.2665537156843864607935756794176995754241943359375;1.2519343893253871424775525156292133033275604248046875;1.6640704536908546007367704078205861151218414306640625;0.98834094938644645456093940083519555628299713134765625;-0.352365830708129046389132099648122675716876983642578125;-0.2108555827386033865167291878606192767620086669921875;-0.93866443787772835261051795896491967141628265380859375;0.093136142442789837669891994664794765412807464599609375]
      mask Display: e = 0.06;c1 = [120 150 230]/255;c2 = ([120 150 230]+0)/383;c3 = ([120 150 230]+128)/383;patch([0 1 1 0],[0 0 1 1],c1);patch([0 1 1 1-e 1-e 0+e],[0 0 1 1-e 0+e 0+e],c2);patch([0 0 1 1-e 0+e 0+e],[0 1 1 1-e 1-e 0+e],c3);plot([0 1 1 0 0],[0 0 1 1 0]);disp('weights');
  "IW{3,2}(6,:)'" : Constant  Value=[-0.540843437218527345322627297719009220600128173828125;-0.9553651906102775814844108026591129601001739501953125;-0.61390389793279764862887759591103531420230865478515625;0.57613097917578992568365947590791620314121246337890625;-1.3194674036138278605534424059442244470119476318359375;0.6447888144472602167667218964197672903537750244140625;-0.036176676120778912537634397494912263937294483184814453125;0.88865513006974861109910079903784207999706268310546875;-0.254267751738635416902667429894790984690189361572265625;0.309308642040444448095826146527542732656002044677734375]
      mask Display: e = 0.06;c1 = [120 150 230]/255;c2 = ([120 150 230]+0)/383;c3 = ([120 150 230]+128)/383;patch([0 1 1 0],[0 0 1 1],c1);patch([0 1 1 1-e 1-e 0+e],[0 0 1 1-e 0+e 0+e],c2);patch([0 0 1 1-e 0+e 0+e],[0 1 1 1-e 1-e 0+e],c3);plot([0 1 1 0 0],[0 0 1 1 0]);disp('weights');
  "IW{3,2}(7,:)'" : Constant  Value=[0.397320906630153292127261011046357452869415283203125;-0.0820837047112922546521218691850663162767887115478515625;0.03454953427473160532112927967318682931363582611083984375;-0.9182898707811915084420206767390482127666473388671875;-0.45957976609613482299465658797998912632465362548828125;0.58337865330045735046127219902700744569301605224609375;-1.5795744374945515087205194504349492490291595458984375;1.0525052175145706012671098505961708724498748779296875;-0.2115172316479299041702688555233180522918701171875;-0.326766824236371211664931024643010459840297698974609375]
      mask Display: e = 0.06;c1 = [120 150 230]/255;c2 = ([120 150 230]+0)/383;c3 = ([120 150 230]+128)/383;patch([0 1 1 0],[0 0 1 1],c1);patch([0 1 1 1-e 1-e 0+e],[0 0 1 1-e 0+e 0+e],c2);patch([0 0 1 1-e 0+e 0+e],[0 1 1 1-e 1-e 0+e],c3);plot([0 1 1 0 0],[0 0 1 1 0]);disp('weights');
  "IW{3,2}(8,:)'" : Constant  Value=[-1.24444177561713598123560586827807128429412841796875;0.86460812239970163961544358244282193481922149658203125;-0.69941815860917255776030287961475551128387451171875;1.1812911486715853559559263885603286325931549072265625;-0.12104072417785140258761344966842443682253360748291015625;-2.4817754822556850058390409685671329498291015625;0.52528013081170288334220686010667122900485992431640625;-0.1853838723087704865033487067194073460996150970458984375;0.2009537471011579035096161760520772077143192291259765625;0.89222319293706731091475603534490801393985748291015625]
      mask Display: e = 0.06;c1 = [120 150 230]/255;c2 = ([120 150 230]+0)/383;c3 = ([120 150 230]+128)/383;patch([0 1 1 0],[0 0 1 1],c1);patch([0 1 1 1-e 1-e 0+e],[0 0 1 1-e 0+e 0+e],c2);patch([0 0 1 1-e 0+e 0+e],[0 1 1 1-e 1-e 0+e],c3);plot([0 1 1 0 0],[0 0 1 1 0]);disp('weights');
  "IW{3,2}(9,:)'" : Constant  Value=[0.023104259103925377238919480760159785859286785125732421875;-0.10292723972935786946880654113556374795734882354736328125;-0.29996084832531588748594231219612993299961090087890625;-1.0195042845657431573869189378456212580204010009765625;-2.59146083484989286915833872626535594463348388671875;1.5301144992831512414710459779598750174045562744140625;-1.76325742159056186864063420216552913188934326171875;0.45101906711502504077060393683495931327342987060546875;0.234305533924234643539108446930185891687870025634765625;-0.66788764273996170661717997063533402979373931884765625]
      mask Display: e = 0.06;c1 = [120 150 230]/255;c2 = ([120 150 230]+0)/383;c3 = ([120 150 230]+128)/383;patch([0 1 1 0],[0 0 1 1],c1);patch([0 1 1 1-e 1-e 0+e],[0 0 1 1-e 0+e 0+e],c2);patch([0 0 1 1-e 0+e 0+e],[0 1 1 1-e 1-e 0+e],c3);plot([0 1 1 0 0],[0 0 1 1 0]);disp('weights');
  Mux : Mux  Inputs=10
      mask Display: e = 0.06;c1 = [120 150 230]/255;c2 = ([120 150 230]+0)/383;c3 = ([120 150 230]+128)/383;patch([0 1 1 0],[0 0 1 1],c1);patch([0 1 1 1-e 1-e 0+e],[0 0 1 1-e 0+e 0+e],c2);patch([0 0 1 1-e 0+e 0+e],[0 1 1 1-e 1-e 0+e],c3);plot([0 1 1 0 0],[0 0 1 1 0]);disp('Mux');
  dotprod{1..10} (10 alike) : neural/Weight Functions/dotprod
  "lz{3,2}" : Outport
      mask Display: e = 0.06;c1 = [120 230 180]/255;c2 = ([120 230 180]+0)/(256+128);c3 = ([120 230 180]+128)/(256+128);patch([0 1 1 0],[0 0 1 1],c1);patch([0 1 1 1-e 1-e 0+e],[0 0 1 1-e 0+e 0+e],c2);patch([0 0 1 1-e 0+e 0+e],[0 1 1 1-e 1-e 0+e],c3);plot([0 1 1 0 0],[0 0 1 1 0]);
  wires:
  "IW{3,2}(1,:)'"/1 -> dotprod1/1
  "ad{3,2}"/1 -> dotprod1/2, dotprod2/2, dotprod3/2, dotprod4/2, dotprod5/2, dotprod6/2, dotprod7/2, dotprod8/2, dotprod9/2, dotprod10/2
  dotprod1/1 -> Mux/1
  "IW{3,2}(2,:)'"/1 -> dotprod2/1
  dotprod2/1 -> Mux/2
  "IW{3,2}(3,:)'"/1 -> dotprod3/1
  dotprod3/1 -> Mux/3
  "IW{3,2}(4,:)'"/1 -> dotprod4/1
  dotprod4/1 -> Mux/4
  "IW{3,2}(5,:)'"/1 -> dotprod5/1
  dotprod5/1 -> Mux/5
  "IW{3,2}(6,:)'"/1 -> dotprod6/1
  dotprod6/1 -> Mux/6
  "IW{3,2}(7,:)'"/1 -> dotprod7/1
  dotprod7/1 -> Mux/7
  "IW{3,2}(8,:)'"/1 -> dotprod8/1
  dotprod8/1 -> Mux/8
  "IW{3,2}(9,:)'"/1 -> dotprod9/1
  dotprod9/1 -> Mux/9
  "IW{3,2}(10,:)'"/1 -> dotprod10/1
  dotprod10/1 -> Mux/10
  Mux/1 -> "lz{3,2}"/1

== system ackerman_ROS_neural_controller_v2/1/Layer 4/Delays 1 ==
  "p{4}" : Inport  PortDimensions=10  SampleTime=0.1
      mask Display: e = 0.06;c1 = [120 230 180]/255;c2 = ([120 230 180]+0)/(256+128);c3 = ([120 230 180]+128)/(256+128);patch([0 1 1 0],[0 0 1 1],c1);patch([0 1 1 1-e 1-e 0+e],[0 0 1 1-e 0+e 0+e],c2);patch([0 0 1 1-e 0+e 0+e],[0 1 1 1-e 1-e 0+e],c3);plot([0 1 1 0 0],[0 0 1 1 0]);
  mux : Mux  Inputs=1
      mask Display: e = 0.06;c1 = [120 150 230]/255;c2 = ([120 150 230]+0)/383;c3 = ([120 150 230]+128)/383;patch([0 1 1 0],[0 0 1 1],c1);patch([0 1 1 1-e 1-e 0+e],[0 0 1 1-e 0+e 0+e],c2);patch([0 0 1 1-e 0+e 0+e],[0 1 1 1-e 1-e 0+e],c3);plot([0 1 1 0 0],[0 0 1 1 0]);disp('Mux')
  "pd{4,3}" : Outport
      mask Display: e = 0.06;c1 = [120 230 180]/255;c2 = ([120 230 180]+0)/(256+128);c3 = ([120 230 180]+128)/(256+128);patch([0 1 1 0],[0 0 1 1],c1);patch([0 1 1 1-e 1-e 0+e],[0 0 1 1-e 0+e 0+e],c2);patch([0 0 1 1-e 0+e 0+e],[0 1 1 1-e 1-e 0+e],c3);plot([0 1 1 0 0],[0 0 1 1 0]);
  wires:
  "p{4}"/1 -> mux/1
  mux/1 -> "pd{4,3}"/1
